simulink model "PID_GpOrden1_tm1000ms_12V_3kHz"  (Simulink 7.5)
settings: Solver=ode45  StartTime=0.0  StopTime=2500  RelTol=1e-3
settings Model: Creator=Paulo  LastModifiedBy=Paulo

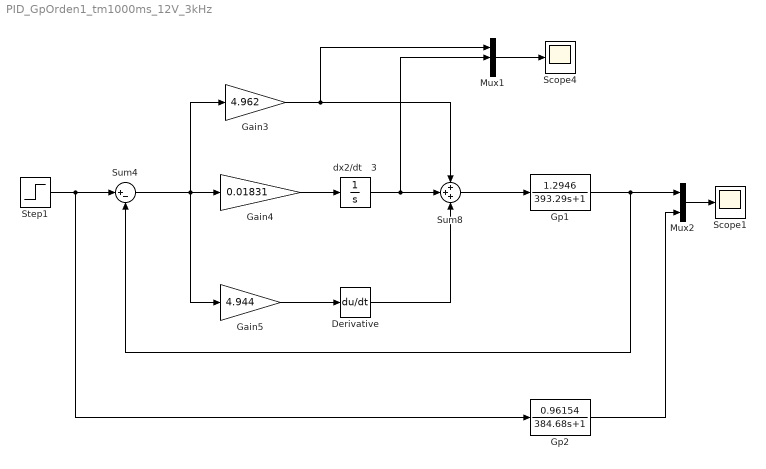
== system PID_GpOrden1_tm1000ms_12V_3kHz ==
  Derivative : Derivative  LinearizePole=100
  Gain3 : Gain  Gain=4.962  ParameterDataType=fixdt(1, 16)  ParameterScaling=2^0  OutDataType=fixdt(1, 16)  OutScaling=2^0
  Gain4 : Gain  Gain=0.01831  ParameterDataType=fixdt(1, 16)  ParameterScaling=2^0  OutDataType=fixdt(1, 16)  OutScaling=2^0
  Gain5 : Gain  Gain=4.944  ParameterDataType=fixdt(1, 16)  ParameterScaling=2^0  OutDataType=fixdt(1, 16)  OutScaling=2^0
  Gp1 : TransferFcn  Numerator=[1.2946]  Denominator=[393.29 1]
  Gp2 : TransferFcn  Numerator=[0.96154]  Denominator=[384.68 1]
  Mux1 : Mux  Inputs=3
  Mux2 : Mux  Inputs=2
  Scope1 : Scope
      settings: TimeRange=10  YMin=-6e+007  YMax=4e+007
  Scope4 : Scope
      settings: TimeRange=10  YMin=-6e+007  YMax=4e+007
  Step1 : Step  SampleTime=0
  Sum4 : Sum  Inputs=|+-  OutDataType=fixdt(1, 16)  OutScaling=2^0
  Sum8 : Sum  Inputs=+++  OutDataType=fixdt(1, 16)  OutScaling=2^0
  dx2/dt   3 : Integrator
  wires:
  Gain3/1 -> Sum8/1, Mux1/1
  Sum4/1 -> Gain3/1, Gain4/1, Gain5/1
  Mux1/1 -> Scope4/1
  Sum8/1 -> Gp1/1
  Gain5/1 -> Derivative/1
  Gain4/1 -> dx2/dt   3/1
  Step1/1 -> Sum4/1, Gp2/1
  Gp1/1 -> Sum4/2, Mux2/1
  dx2/dt   3/1 -> Sum8/2, Mux1/2
  Mux2/1 -> Scope1/1
  Gp2/1 -> Mux2/2
  Derivative/1 -> Sum8/3
